simulink library "halout"  (R2021b)
settings: Solver=VariableStepAuto  StartTime=0.0  StopTime=10.0  RelTol=1e-3
undefined symbols (not defined in the file): C_TASK_5MS_S, FALSE, KHAL_CAN1TxReq_flg, KHAL_CAN2TxReq_flg, KHAL_CAN3FD3VCU1toNIDECTxReq_flg, KHAL_CAN3FD3VCU1TxReq_flg, KHAL_CAN3FD3VCU2E2E_flg, KHAL_CAN3FD3VCU2toNIDECE2E_flg, KHAL_CAN3FD3VCU2toNIDECTxReq_flg, KHAL_CAN3FD3VCU2TxReq_flg, KHAL_CAN3TxReq_flg, KHAL_CAN4FD4CE1000E2E_flg, KHAL_CAN4FD4CE1000TxReq_flg, KHAL_CAN4TxReq_flg, KHAL_CAN5TxReq_flg, KHAL_CAN7TxReq_flg, ONE_INT, TRUE, ZERO_INT
libraries: FVT_lib x258, simulink x115
(part 6 of 17)

== system halout/HAL_OUT/CAN3/FD3_VCU1_toNIDEC_0x116 ==
  BSCP_outputs : Inport  OutDataTypeStr=Bus: BSCP_outputs
  BOUTP_outputs : Inport  Port=2  OutDataTypeStr=Bus: BOUTP_outputs
  ActiveDischReqtoNidec : Subsystem
  CSVCU1toNidec : Subsystem
  CoastDwModeStaChktoNidec : Subsystem
  DCDCEnaReqtoNidec : Subsystem
  DCDCVoltSetpointtoNidec : Subsystem
  DemoModeStaChktoNidec : Subsystem
  DrSeatStatoNidec : Subsystem
  DynoModeStaChktoNidec : Subsystem
  FrActvDmpDisabReqtoNidec : Subsystem
  FrMCUEnaReqtoNidec : Subsystem
  Ground{,1..6} (7 alike) : Ground
  HVBatCnctReqtoNidec : Subsystem
  HVSysReadyToChargetoNidec : Subsystem
  LVChrgFuncStaChktoNidec : Subsystem
  MSACrlStatoNidec : Subsystem
  PrkReqtoNidec : Subsystem
  PwrStatoNidec : Subsystem
  RCVCU1toNidec : Subsystem
  RrActvDmpDisabReqtoNidec : Subsystem
  RrMCUEnaReqtoNidec : Subsystem
  ShiftGearPosntoNidec : Subsystem
  bus_creator : BusCreator  Inputs=20  OutDataTypeStr=Bus: DT_CAN3_SG_FD3_VCU1_toNIDEC  NonVirtualBus=on
  bus_selector : BusSelector  OutputSignals=VOUTP_ActiveDischargeReq_flg
  bus_selector1 : BusSelector  OutputSignals=VOUTP_DCDCEnaReq_flg
  bus_selector10 : BusSelector  OutputSignals=VOUTP_RrActvDmpDisabReq_flg
  bus_selector11 : BusSelector  OutputSignals=VOUTP_RrMCUEnaReq_flg
  bus_selector12 : BusSelector  OutputSignals=VOUTP_ShiftGearPosn_enum
  bus_selector2 : BusSelector  OutputSignals=VOUTP_DCDCVoltSetpoint_V
  bus_selector3 : BusSelector  OutputSignals=VOUTP_DrSeatSta_enum
  bus_selector4 : BusSelector  OutputSignals=VOUTP_FrActvDmpDisabReq_flg
  bus_selector5 : BusSelector  OutputSignals=VOUTP_FrMCUEnaReq_flg
  bus_selector6 : BusSelector  OutputSignals=VOUTP_HVBatCnctReq_flg
  bus_selector7 : BusSelector  OutputSignals=VOUTP_HVSysReadyToCharge_enum
  bus_selector8 : BusSelector  OutputSignals=VOUTP_MSACtrlSta_enum
  bus_selector9 : BusSelector  OutputSignals=VOUTP_PowerSta_enum
  FD3_VCU1_toNIDEC : Outport
  wires:
  BSCP_outputs/1 -> [BSCP_outputs]
  BOUTP_outputs/1 -> [BOUTP_outputs]
  [CAN3_ActiveDischReq_toNidec] -> bus_creator/1  "CAN3_ActiveDischReq_toNidec"
  [CAN3_CS_VCU1_toNidec] -> bus_creator/2  "CAN3_CS_VCU1_toNidec"
  [CAN3_CoastDwModeStaChk_toNidec] -> bus_creator/3  "CAN3_CoastDwModeStaChk_toNidec"
  [CAN3_DCDCEnaReq_toNidec] -> bus_creator/4  "CAN3_DCDCEnaReq_toNidec"
  [CAN3_DCDCVoltSetpoint_toNidec] -> bus_creator/5  "CAN3_DCDCVoltSetpoint_toNidec"
  [CAN3_DemoModeStaChk_toNidec] -> bus_creator/6  "CAN3_DemoModeStaChk_toNidec"
  [CAN3_Dr_SeatSta_toNidec] -> bus_creator/7  "CAN3_Dr_SeatSta_toNidec"
  [CAN3_DynoModeStaChk_toNidec] -> bus_creator/8  "CAN3_DynoModeStaChk_toNidec"
  [CAN3_Fr_ActvDmpDisabReq_toNidec] -> bus_creator/9  "CAN3_Fr_ActvDmpDisabReq_toNidec"
  [CAN3_Fr_MCUEnaReq_toNidec] -> bus_creator/10  "CAN3_Fr_MCUEnaReq_toNidec"
  [CAN3_HVBatCnctReq_toNidec] -> bus_creator/11  "CAN3_HVBatCnctReq_toNidec"
  [CAN3_HVSysReadyToCharge_toNidec] -> bus_creator/12  "CAN3_HVSysReadyToCharge_toNidec"
  [CAN3_LVChrgFuncStaChk_toNidec] -> bus_creator/13  "CAN3_LVChrgFuncStaChk_toNidec"
  [CAN3_MSA_Crl_Sta_toNidec] -> bus_creator/14  "CAN3_MSA_Crl_Sta_toNidec"
  [CAN3_PrkReq_toNidec] -> bus_creator/15  "CAN3_PrkReq_toNidec"
  [CAN3_PwrSta_toNidec] -> bus_creator/16  "CAN3_PwrSta_toNidec"
  [CAN3_RC_VCU1_toNidec] -> bus_creator/17  "CAN3_RC_VCU1_toNidec"
  [CAN3_Rr_ActvDmpDisabReq_toNidec] -> bus_creator/18  "CAN3_Rr_ActvDmpDisabReq_toNidec"
  [CAN3_Rr_MCUEnaReq_toNidec] -> bus_creator/19  "CAN3_Rr_MCUEnaReq_toNidec"
  [CAN3_ShiftGearPosn_toNidec] -> bus_creator/20  "CAN3_ShiftGearPosn_toNidec"
  bus_creator/1 -> FD3_VCU1_toNIDEC/1
  ActiveDischReqtoNidec/1(CAN3_ActiveDischReq_toNidec) -> [CAN3_ActiveDischReq_toNidec]
  CSVCU1toNidec/1(CAN3_CS_VCU1_toNidec) -> [CAN3_CS_VCU1_toNidec]
  CoastDwModeStaChktoNidec/1(CAN3_CoastDwModeStaChk_toNidec) -> [CAN3_CoastDwModeStaChk_toNidec]
  DCDCEnaReqtoNidec/1(CAN3_DCDCEnaReq_toNidec) -> [CAN3_DCDCEnaReq_toNidec]
  DCDCVoltSetpointtoNidec/1(CAN3_DCDCVoltSetpoint_toNidec) -> [CAN3_DCDCVoltSetpoint_toNidec]
  DemoModeStaChktoNidec/1(CAN3_DemoModeStaChk_toNidec) -> [CAN3_DemoModeStaChk_toNidec]
  DrSeatStatoNidec/1(CAN3_Dr_SeatSta_toNidec) -> [CAN3_Dr_SeatSta_toNidec]
  DynoModeStaChktoNidec/1(CAN3_DynoModeStaChk_toNidec) -> [CAN3_DynoModeStaChk_toNidec]
  FrActvDmpDisabReqtoNidec/1(CAN3_Fr_ActvDmpDisabReq_toNidec) -> [CAN3_Fr_ActvDmpDisabReq_toNidec]
  FrMCUEnaReqtoNidec/1(CAN3_Fr_MCUEnaReq_toNidec) -> [CAN3_Fr_MCUEnaReq_toNidec]
  HVBatCnctReqtoNidec/1(CAN3_HVBatCnctReq_toNidec) -> [CAN3_HVBatCnctReq_toNidec]
  HVSysReadyToChargetoNidec/1(CAN3_HVSysReadyToCharge_toNidec) -> [CAN3_HVSysReadyToCharge_toNidec]
  LVChrgFuncStaChktoNidec/1(CAN3_LVChrgFuncStaChk_toNidec) -> [CAN3_LVChrgFuncStaChk_toNidec]
  MSACrlStatoNidec/1(CAN3_MSA_Crl_Sta_toNidec) -> [CAN3_MSA_Crl_Sta_toNidec]
  PrkReqtoNidec/1(CAN3_PrkReq_toNidec) -> [CAN3_PrkReq_toNidec]
  PwrStatoNidec/1(CAN3_PwrSta_toNidec) -> [CAN3_PwrSta_toNidec]
  RCVCU1toNidec/1(CAN3_RC_VCU1_toNidec) -> [CAN3_RC_VCU1_toNidec]
  RrActvDmpDisabReqtoNidec/1(CAN3_Rr_ActvDmpDisabReq_toNidec) -> [CAN3_Rr_ActvDmpDisabReq_toNidec]
  RrMCUEnaReqtoNidec/1(CAN3_Rr_MCUEnaReq_toNidec) -> [CAN3_Rr_MCUEnaReq_toNidec]
  ShiftGearPosntoNidec/1(CAN3_ShiftGearPosn_toNidec) -> [CAN3_ShiftGearPosn_toNidec]
  bus_selector/1 -> ActiveDischReqtoNidec/1(ActiveDischReqtoNidec)  "<VOUTP_ActiveDischargeReq_flg>"
  [BOUTP_outputs] -> bus_selector/1
  Ground/1 -> CSVCU1toNidec/1(CSVCU1toNidec)
  Ground1/1 -> CoastDwModeStaChktoNidec/1(CoastDwModeStaChktoNidec)
  bus_selector1/1 -> DCDCEnaReqtoNidec/1(DCDCEnaReqtoNidec)  "<VOUTP_DCDCEnaReq_flg>"
  [BOUTP_outputs] -> bus_selector1/1
  bus_selector2/1 -> DCDCVoltSetpointtoNidec/1(DCDCVoltSetpointtoNidec)  "<VOUTP_DCDCVoltSetpoint_V>"
  [BOUTP_outputs] -> bus_selector2/1
  Ground2/1 -> DemoModeStaChktoNidec/1(DemoModeStaChktoNidec)
  bus_selector3/1 -> DrSeatStatoNidec/1(DrSeatStatoNidec)  "<VOUTP_DrSeatSta_enum>"
  [BOUTP_outputs] -> bus_selector3/1
  Ground3/1 -> DynoModeStaChktoNidec/1(DynoModeStaChktoNidec)
  bus_selector4/1 -> FrActvDmpDisabReqtoNidec/1(FrActvDmpDisabReqtoNidec)  "<VOUTP_FrActvDmpDisabReq_flg>"
  [BOUTP_outputs] -> bus_selector4/1
  bus_selector5/1 -> FrMCUEnaReqtoNidec/1(FrMCUEnaReqtoNidec)  "<VOUTP_FrMCUEnaReq_flg>"
  [BOUTP_outputs] -> bus_selector5/1
  bus_selector6/1 -> HVBatCnctReqtoNidec/1(HVBatCnctReqtoNidec)  "<VOUTP_HVBatCnctReq_flg>"
  [BOUTP_outputs] -> bus_selector6/1
  bus_selector7/1 -> HVSysReadyToChargetoNidec/1(HVSysReadyToChargetoNidec)  "<VOUTP_HVSysReadyToCharge_enum>"
  [BOUTP_outputs] -> bus_selector7/1
  Ground4/1 -> LVChrgFuncStaChktoNidec/1(LVChrgFuncStaChktoNidec)
  bus_selector8/1 -> MSACrlStatoNidec/1(MSACrlStatoNidec)  "<VOUTP_MSACtrlSta_enum>"
  [BOUTP_outputs] -> bus_selector8/1
  Ground5/1 -> PrkReqtoNidec/1(PrkReqtoNidec)
  bus_selector9/1 -> PwrStatoNidec/1(PwrStatoNidec)  "<VOUTP_PowerSta_enum>"
  [BOUTP_outputs] -> bus_selector9/1
  Ground6/1 -> RCVCU1toNidec/1(RCVCU1toNidec)
  bus_selector10/1 -> RrActvDmpDisabReqtoNidec/1(RrActvDmpDisabReqtoNidec)  "<VOUTP_RrActvDmpDisabReq_flg>"
  [BOUTP_outputs] -> bus_selector10/1
  bus_selector11/1 -> RrMCUEnaReqtoNidec/1(RrMCUEnaReqtoNidec)  "<VOUTP_RrMCUEnaReq_flg>"
  [BOUTP_outputs] -> bus_selector11/1
  bus_selector12/1 -> ShiftGearPosntoNidec/1(ShiftGearPosntoNidec)  "<VOUTP_ShiftGearPosn_enum>"
  [BOUTP_outputs] -> bus_selector12/1

== system halout/HAL_OUT/CAN3/FD3_VCU1_toNIDEC_Tx ==
  TxReq : Inport
  BSCP_outputs : Inport  Port=2  OutDataTypeStr=Bus: BSCP_outputs
  BOUTP_outputs : Inport  Port=3  OutDataTypeStr=Bus: BOUTP_outputs
  Chart : Stateflow chart  AncestorBlock=haloutREF/HAL_OUT/CAN3/FD3_VCU1_toNIDEC_Tx/Chart  TreatAsAtomicUnit=on
  Constant : Constant  Value=C_TASK_5MS_S
  Constant3 : Constant  Value=CycleTime
  Data Type Conversion : DataTypeConversion  OutDataTypeStr=uint16
  Data Type Conversion1 : DataTypeConversion  OutDataTypeStr=uint8
  Divide : Product  Inputs=*/
  Gain : Gain  Gain=0.001
  Ground{,1..6} (7 alike) : Ground
  OR : Logic  Operator=OR  Inputs=20  AllPortsSameDT=off  OutDataTypeStr=boolean
  bus_selector : BusSelector  OutputSignals=VOUTP_ActiveDischargeReq_flg
  bus_selector1 : BusSelector  OutputSignals=VOUTP_DCDCEnaReq_flg
  bus_selector10 : BusSelector  OutputSignals=VOUTP_RrActvDmpDisabReq_flg
  bus_selector11 : BusSelector  OutputSignals=VOUTP_RrMCUEnaReq_flg
  bus_selector12 : BusSelector  OutputSignals=VOUTP_ShiftGearPosn_enum
  bus_selector2 : BusSelector  OutputSignals=VOUTP_DCDCVoltSetpoint_V
  bus_selector3 : BusSelector  OutputSignals=VOUTP_DrSeatSta_enum
  bus_selector4 : BusSelector  OutputSignals=VOUTP_FrActvDmpDisabReq_flg
  bus_selector5 : BusSelector  OutputSignals=VOUTP_FrMCUEnaReq_flg
  bus_selector6 : BusSelector  OutputSignals=VOUTP_HVBatCnctReq_flg
  bus_selector7 : BusSelector  OutputSignals=VOUTP_HVSysReadyToCharge_enum
  bus_selector8 : BusSelector  OutputSignals=VOUTP_MSACtrlSta_enum
  bus_selector9 : BusSelector  OutputSignals=VOUTP_PowerSta_enum
  convert_out : FVT_lib/hal/convert_out  gain=0.0235  offset=12
  detect_change{,1..12} (13 alike) : simulink/Logic and Bit Operations/Detect Change  vinit=0  OutDataTypeStr=boolean
  TxTrigger : Outport
  wires:
  Data Type Conversion/1 -> Chart/3(CycleCnt)
  TxReq/1 -> Chart/1(TxReq)
  [EventReq_flg] -> Chart/2(EventReq)
  Constant/1 -> Divide/2
  Divide/1 -> Data Type Conversion/1
  Chart/1(TxTrigger) -> TxTrigger/1
  Gain/1 -> Divide/1
  Constant3/1 -> Gain/1
  BSCP_outputs/1 -> [BSCP_outputs]
  BOUTP_outputs/1 -> [BOUTP_outputs]
  OR/1 -> [EventReq_flg]
  detect_change/1 -> OR/1
  bus_selector/1 -> detect_change/1  "<VOUTP_ActiveDischargeReq_flg>"
  [BOUTP_outputs] -> bus_selector/1
  Ground/1 -> OR/2
  Ground1/1 -> OR/3
  detect_change1/1 -> OR/4
  bus_selector1/1 -> detect_change1/1  "<VOUTP_DCDCEnaReq_flg>"
  [BOUTP_outputs] -> bus_selector1/1
  detect_change2/1 -> OR/5
  Data Type Conversion1/1 -> detect_change2/1
  convert_out/1 -> Data Type Conversion1/1
  bus_selector2/1 -> convert_out/1  "<VOUTP_DCDCVoltSetpoint_V>"
  [BOUTP_outputs] -> bus_selector2/1
  Ground2/1 -> OR/6
  detect_change3/1 -> OR/7
  bus_selector3/1 -> detect_change3/1  "<VOUTP_DrSeatSta_enum>"
  [BOUTP_outputs] -> bus_selector3/1
  Ground3/1 -> OR/8
  detect_change4/1 -> OR/9
  bus_selector4/1 -> detect_change4/1  "<VOUTP_FrActvDmpDisabReq_flg>"
  [BOUTP_outputs] -> bus_selector4/1
  detect_change5/1 -> OR/10
  bus_selector5/1 -> detect_change5/1  "<VOUTP_FrMCUEnaReq_flg>"
  [BOUTP_outputs] -> bus_selector5/1
  detect_change6/1 -> OR/11
  bus_selector6/1 -> detect_change6/1  "<VOUTP_HVBatCnctReq_flg>"
  [BOUTP_outputs] -> bus_selector6/1
  detect_change7/1 -> OR/12
  bus_selector7/1 -> detect_change7/1  "<VOUTP_HVSysReadyToCharge_enum>"
  [BOUTP_outputs] -> bus_selector7/1
  Ground4/1 -> OR/13
  detect_change8/1 -> OR/14
  bus_selector8/1 -> detect_change8/1  "<VOUTP_MSACtrlSta_enum>"
  [BOUTP_outputs] -> bus_selector8/1
  Ground5/1 -> OR/15
  detect_change9/1 -> OR/16
  bus_selector9/1 -> detect_change9/1  "<VOUTP_PowerSta_enum>"
  [BOUTP_outputs] -> bus_selector9/1
  Ground6/1 -> OR/17
  detect_change10/1 -> OR/18
  bus_selector10/1 -> detect_change10/1  "<VOUTP_RrActvDmpDisabReq_flg>"
  [BOUTP_outputs] -> bus_selector10/1
  detect_change11/1 -> OR/19
  bus_selector11/1 -> detect_change11/1  "<VOUTP_RrMCUEnaReq_flg>"
  [BOUTP_outputs] -> bus_selector11/1
  detect_change12/1 -> OR/20
  bus_selector12/1 -> detect_change12/1  "<VOUTP_ShiftGearPosn_enum>"
  [BOUTP_outputs] -> bus_selector12/1

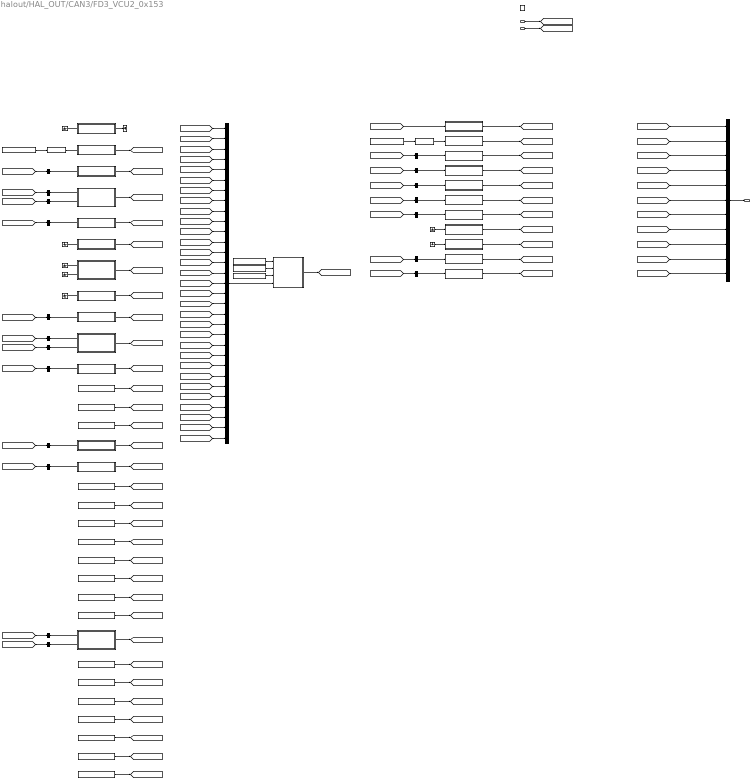
== system halout/HAL_OUT/CAN3/FD3_VCU2_0x153 ==
  BSCP_outputs : Inport  OutDataTypeStr=Bus: BSCP_outputs
  BOUTP_outputs : Inport  Port=2  OutDataTypeStr=Bus: BOUTP_outputs
  Trigger : TriggerPort  TriggerType=function-call  VariantControl=(inherit)
  Byte_0 : Subsystem
  Byte_1 : Subsystem
  Byte_10 : Subsystem
  Byte_{11..13,16..23,25..31} (18 alike) : Constant  Value=ZERO_INT
  Byte_14 : Subsystem
  Byte_15 : Subsystem
  Byte_2 : Subsystem
  Byte_24 : Subsystem
  Byte_3 : Subsystem
  Byte_4 : Subsystem
  Byte_5 : Subsystem
  Byte_6 : Subsystem
  Byte_7 : Subsystem
  Byte_8 : Subsystem
  Byte_9 : Subsystem
  CRC8_IfAction_Tx : Subsystem  AncestorBlock=FVT_lib/hal/CRC8_IfAction_Tx
      mask help: MeasumentTrigerEvent
      mask Display: fprintf('CRC8_IfAction');
  CSVCU2CAN1 : Subsystem
  Constant : Constant  Value=KHAL_CAN3FD3VCU2E2E_flg
  Constant1 : Constant  Value=0x40
  Constant2 : Constant  Value=0x24
  Constant3 : Constant  Value=KHAL_CAN3FD3VCU2E2E_flg
  Constant4 : Constant  Value=KHAL_CAN3FD3VCU2E2E_flg
  Ground{,1..6} (7 alike) : Ground
  Mux2 : Mux  Inputs=31
  RCVCU2CAN1 : Subsystem
  RollingCounter_IfAction : FVT_lib/hal/RollingCounter_IfAction
  RollingCounter_IfAction1 : FVT_lib/hal/RollingCounter_IfAction
  RrActvDmpDisabReq : Subsystem
  RrIdcMax : Subsystem
  RrIdcMin : Subsystem
  RrMCUEnaReq : Subsystem
  RrTMTqReq : Subsystem
  RrTorqMax : Subsystem
  RrTorqMin : Subsystem
  RrUdcMax : Subsystem
  RrUdcMin : Subsystem
  Terminator : Terminator
  bus_creator : BusCreator  Inputs=11  OutDataTypeStr=Bus: DT_CAN3_SG_FD3_VCU2  NonVirtualBus=on
  bus_selector : BusSelector  OutputSignals=VOUTP_RrIdcMax_A
  bus_selector1 : BusSelector  OutputSignals=VOUTP_RrIdcMax_A
  bus_selector10 : BusSelector  OutputSignals=VOUTP_RrActvDmpDisabReq_flg
  bus_selector11 : BusSelector  OutputSignals=VOUTP_RrMCUEnaReq_flg
  bus_selector12 : BusSelector  OutputSignals=VOUTP_RrActvDmpDisabReq_flg
  bus_selector13 : BusSelector  OutputSignals=VOUTP_RrIdcMax_A
  bus_selector14 : BusSelector  OutputSignals=VOUTP_RrIdcMin_A
  bus_selector15 : BusSelector  OutputSignals=VOUTP_RrMCUEnaReq_flg
  bus_selector16 : BusSelector  OutputSignals=VOUTP_RrTMTqReq_Nm
  bus_selector17 : BusSelector  OutputSignals=VOUTP_RrUdcMax_V
  bus_selector18 : BusSelector  OutputSignals=VOUTP_RrUdcMin_V
  bus_selector2 : BusSelector  OutputSignals=VOUTP_RrIdcMin_A
  bus_selector3 : BusSelector  OutputSignals=VOUTP_RrIdcMin_A
  bus_selector4 : BusSelector  OutputSignals=VOUTP_RrUdcMax_V
  bus_selector5 : BusSelector  OutputSignals=VOUTP_RrUdcMax_V
  bus_selector6 : BusSelector  OutputSignals=VOUTP_RrUdcMin_V
  bus_selector7 : BusSelector  OutputSignals=VOUTP_RrUdcMin_V
  bus_selector8 : BusSelector  OutputSignals=VOUTP_RrTMTqReq_Nm
  bus_selector9 : BusSelector  OutputSignals=VOUTP_RrTMTqReq_Nm
  FD3_VCU2 : Outport
  wires:
  BSCP_outputs/1 -> [BSCP_outputs]
  BOUTP_outputs/1 -> [BOUTP_outputs]
  [CAN3_CS_VCU2_CAN1] -> bus_creator/1  "CAN3_CS_VCU2_CAN1"
  [CAN3_RC_VCU2_CAN1] -> bus_creator/2  "CAN3_RC_VCU2_CAN1"
  [CAN3_Rr_ActvDmpDisabReq] -> bus_creator/3  "CAN3_Rr_ActvDmpDisabReq"
  [CAN3_Rr_IdcMax] -> bus_creator/4  "CAN3_Rr_IdcMax"
  [CAN3_Rr_IdcMin] -> bus_creator/5  "CAN3_Rr_IdcMin"
  [CAN3_Rr_MCUEnaReq] -> bus_creator/6  "CAN3_Rr_MCUEnaReq"
  [CAN3_Rr_TMTqReq] -> bus_creator/7  "CAN3_Rr_TMTqReq"
  [CAN3_Rr_TorqMax] -> bus_creator/8  "CAN3_Rr_TorqMax"
  [CAN3_Rr_TorqMin] -> bus_creator/9  "CAN3_Rr_TorqMin"
  [CAN3_Rr_UdcMax] -> bus_creator/10  "CAN3_Rr_UdcMax"
  [CAN3_Rr_UdcMin] -> bus_creator/11  "CAN3_Rr_UdcMin"
  bus_creator/1 -> FD3_VCU2/1
  CSVCU2CAN1/1(CAN3_CS_VCU2_CAN1) -> [CAN3_CS_VCU2_CAN1]
  RCVCU2CAN1/1(CAN3_RC_VCU2_CAN1) -> [CAN3_RC_VCU2_CAN1]
  RrActvDmpDisabReq/1(CAN3_Rr_ActvDmpDisabReq) -> [CAN3_Rr_ActvDmpDisabReq]
  RrIdcMax/1(CAN3_Rr_IdcMax) -> [CAN3_Rr_IdcMax]
  RrIdcMin/1(CAN3_Rr_IdcMin) -> [CAN3_Rr_IdcMin]
  RrMCUEnaReq/1(CAN3_Rr_MCUEnaReq) -> [CAN3_Rr_MCUEnaReq]
  RrTMTqReq/1(CAN3_Rr_TMTqReq) -> [CAN3_Rr_TMTqReq]
  RrTorqMax/1(CAN3_Rr_TorqMax) -> [CAN3_Rr_TorqMax]
  RrTorqMin/1(CAN3_Rr_TorqMin) -> [CAN3_Rr_TorqMin]
  RrUdcMax/1(CAN3_Rr_UdcMax) -> [CAN3_Rr_UdcMax]
  RrUdcMin/1(CAN3_Rr_UdcMin) -> [CAN3_Rr_UdcMin]
  Byte_0/1(Byte_0) -> Terminator/1
  Byte_1/1(Byte_1) -> [Byte_1]
  Byte_2/1(Byte_2) -> [Byte_2]
  Byte_3/1(Byte_3) -> [Byte_3]
  Byte_4/1(Byte_4) -> [Byte_4]
  Byte_5/1(Byte_5) -> [Byte_5]
  Byte_6/1(Byte_6) -> [Byte_6]
  Byte_7/1(Byte_7) -> [Byte_7]
  Byte_8/1(Byte_8) -> [Byte_8]
  Byte_9/1(Byte_9) -> [Byte_9]
  Byte_10/1(Byte_10) -> [Byte_10]
  Byte_11/1 -> [Byte_11]
  Byte_12/1 -> [Byte_12]
  Byte_13/1 -> [Byte_13]
  Byte_14/1(Byte_14) -> [Byte_14]
  Byte_15/1(Byte_15) -> [Byte_15]
  Byte_16/1 -> [Byte_16]
  Byte_17/1 -> [Byte_17]
  Byte_18/1 -> [Byte_18]
  Byte_19/1 -> [Byte_19]
  Byte_20/1 -> [Byte_20]
  Byte_21/1 -> [Byte_21]
  Byte_22/1 -> [Byte_22]
  Byte_23/1 -> [Byte_23]
  Byte_24/1(Byte_24) -> [Byte_24]
  Byte_25/1 -> [Byte_25]
  Byte_26/1 -> [Byte_26]
  Byte_27/1 -> [Byte_27]
  Byte_28/1 -> [Byte_28]
  Byte_29/1 -> [Byte_29]
  Byte_30/1 -> [Byte_30]
  Byte_31/1 -> [Byte_31]
  Mux2/1 -> CRC8_IfAction_Tx/4(RawData)
  Constant/1 -> CRC8_IfAction_Tx/1(CAN_E2E_flg)
  Constant1/1 -> CRC8_IfAction_Tx/2(DataID1)
  Constant2/1 -> CRC8_IfAction_Tx/3(DataID2)
  CRC8_IfAction_Tx/1(CRC8) -> [CS_VCU2_CAN1]
  Ground/1 -> Byte_0/1(CS_VCU2_CAN1)
  [Byte_1] -> Mux2/1
  RollingCounter_IfAction/1 -> Byte_1/1(RC_VCU2_CAN1)
  Constant3/1 -> RollingCounter_IfAction/1
  [Byte_2] -> Mux2/2
  bus_selector/1 -> Byte_2/1(Rr_IdcMax)  "<VOUTP_RrIdcMax_A>"
  [BOUTP_outputs] -> bus_selector/1
  [Byte_3] -> Mux2/3
  bus_selector1/1 -> Byte_3/1(Rr_IdcMax)  "<VOUTP_RrIdcMax_A>"
  [BOUTP_outputs] -> bus_selector1/1
  bus_selector2/1 -> Byte_3/2(Rr_IdcMin)  "<VOUTP_RrIdcMin_A>"
  [BOUTP_outputs] -> bus_selector2/1
  [Byte_4] -> Mux2/4
  bus_selector3/1 -> Byte_4/1(Rr_IdcMin)  "<VOUTP_RrIdcMin_A>"
  [BOUTP_outputs] -> bus_selector3/1
  [Byte_5] -> Mux2/5
  Ground1/1 -> Byte_5/1(Rr_TorqMax)
  [Byte_6] -> Mux2/6
  Ground2/1 -> Byte_6/1(Rr_TorqMax)
  Ground3/1 -> Byte_6/2(Rr_TorqMin)
  [Byte_7] -> Mux2/7
  Ground4/1 -> Byte_7/1(Rr_TorqMin)
  [Byte_8] -> Mux2/8
  bus_selector4/1 -> Byte_8/1(Rr_UdcMax)  "<VOUTP_RrUdcMax_V>"
  [BOUTP_outputs] -> bus_selector4/1
  [Byte_9] -> Mux2/9
  bus_selector5/1 -> Byte_9/1(Rr_UdcMax)  "<VOUTP_RrUdcMax_V>"
  [BOUTP_outputs] -> bus_selector5/1
  bus_selector6/1 -> Byte_9/2(Rr_UdcMin)  "<VOUTP_RrUdcMin_V>"
  [BOUTP_outputs] -> bus_selector6/1
  [Byte_10] -> Mux2/10
  bus_selector7/1 -> Byte_10/1(Rr_UdcMin)  "<VOUTP_RrUdcMin_V>"
  [BOUTP_outputs] -> bus_selector7/1
  [Byte_11] -> Mux2/11
  [Byte_12] -> Mux2/12
  [Byte_13] -> Mux2/13
  [Byte_14] -> Mux2/14
  bus_selector8/1 -> Byte_14/1(Rr_TMTqReq)  "<VOUTP_RrTMTqReq_Nm>"
  [BOUTP_outputs] -> bus_selector8/1
  [Byte_15] -> Mux2/15
  bus_selector9/1 -> Byte_15/1(Rr_TMTqReq)  "<VOUTP_RrTMTqReq_Nm>"
  [BOUTP_outputs] -> bus_selector9/1
  [Byte_16] -> Mux2/16
  [Byte_17] -> Mux2/17
  [Byte_18] -> Mux2/18
  [Byte_19] -> Mux2/19
  [Byte_20] -> Mux2/20
  [Byte_21] -> Mux2/21
  [Byte_22] -> Mux2/22
  [Byte_23] -> Mux2/23
  [Byte_24] -> Mux2/24
  bus_selector10/1 -> Byte_24/1(Rr_ActvDmpDisabReq)  "<VOUTP_RrActvDmpDisabReq_flg>"
  [BOUTP_outputs] -> bus_selector10/1
  bus_selector11/1 -> Byte_24/2(Rr_MCUEnaReq)  "<VOUTP_RrMCUEnaReq_flg>"
  [BOUTP_outputs] -> bus_selector11/1
  [Byte_25] -> Mux2/25
  [Byte_26] -> Mux2/26
  [Byte_27] -> Mux2/27
  [Byte_28] -> Mux2/28
  [Byte_29] -> Mux2/29
  [Byte_30] -> Mux2/30
  [Byte_31] -> Mux2/31
  [CS_VCU2_CAN1] -> CSVCU2CAN1/1(CSVCU2CAN1)
  RollingCounter_IfAction1/1 -> RCVCU2CAN1/1(RCVCU2CAN1)
  Constant4/1 -> RollingCounter_IfAction1/1
  bus_selector12/1 -> RrActvDmpDisabReq/1(RrActvDmpDisabReq)  "<VOUTP_RrActvDmpDisabReq_flg>"
  [BOUTP_outputs] -> bus_selector12/1
  bus_selector13/1 -> RrIdcMax/1(RrIdcMax)  "<VOUTP_RrIdcMax_A>"
  [BOUTP_outputs] -> bus_selector13/1
  bus_selector14/1 -> RrIdcMin/1(RrIdcMin)  "<VOUTP_RrIdcMin_A>"
  [BOUTP_outputs] -> bus_selector14/1
  bus_selector15/1 -> RrMCUEnaReq/1(RrMCUEnaReq)  "<VOUTP_RrMCUEnaReq_flg>"
  [BOUTP_outputs] -> bus_selector15/1
  bus_selector16/1 -> RrTMTqReq/1(RrTMTqReq)  "<VOUTP_RrTMTqReq_Nm>"
  [BOUTP_outputs] -> bus_selector16/1
  Ground5/1 -> RrTorqMax/1(RrTorqMax)
  Ground6/1 -> RrTorqMin/1(RrTorqMin)
  bus_selector17/1 -> RrUdcMax/1(RrUdcMax)  "<VOUTP_RrUdcMax_V>"
  [BOUTP_outputs] -> bus_selector17/1
  bus_selector18/1 -> RrUdcMin/1(RrUdcMin)  "<VOUTP_RrUdcMin_V>"
  [BOUTP_outputs] -> bus_selector18/1

== system halout/HAL_OUT/CAN3/FD3_VCU2_Tx ==
  TxReq : Inport
  Chart : Stateflow chart  TreatAsAtomicUnit=on
  Constant : Constant  Value=C_TASK_5MS_S
  Constant3 : Constant  Value=CycleTime
  Data Type Conversion : DataTypeConversion  OutDataTypeStr=uint16
  Divide : Product  Inputs=*/
  Gain : Gain  Gain=0.001
  TxTrigger : Outport
  wires:
  Data Type Conversion/1 -> Chart/2(CycleCnt)
  Constant3/1 -> Gain/1
  Gain/1 -> Divide/1
  Chart/1(TxTrigger()) -> TxTrigger/1
  Divide/1 -> Data Type Conversion/1
  TxReq/1 -> Chart/1(TxReq)
  Constant/1 -> Divide/2

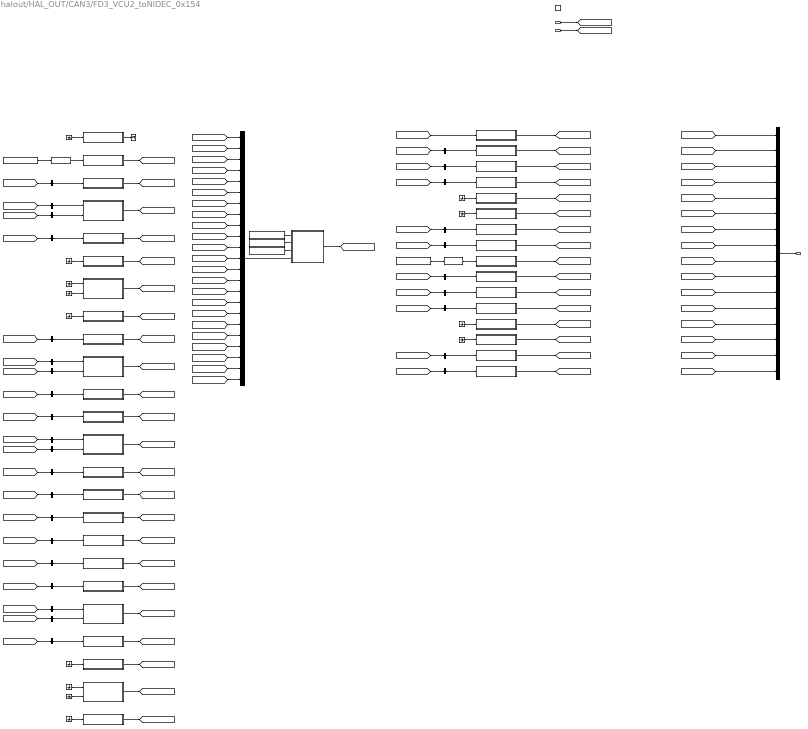
== system halout/HAL_OUT/CAN3/FD3_VCU2_toNIDEC_0x154 ==
  BSCP_outputs : Inport  OutDataTypeStr=Bus: BSCP_outputs
  BOUTP_outputs : Inport  Port=2  OutDataTypeStr=Bus: BOUTP_outputs
  Trigger : TriggerPort  TriggerType=function-call  VariantControl=(inherit)
  Byte_0 : Subsystem
  Byte_1 : Subsystem
  Byte_10 : Subsystem
  Byte_11 : Subsystem
  Byte_12 : Subsystem
  Byte_13 : Subsystem
  Byte_14 : Subsystem
  Byte_15 : Subsystem
  Byte_16 : Subsystem
  Byte_17 : Subsystem
  Byte_18 : Subsystem
  Byte_19 : Subsystem
  Byte_2 : Subsystem
  Byte_20 : Subsystem
  Byte_21 : Subsystem
  Byte_22 : Subsystem
  Byte_23 : Subsystem
  Byte_3 : Subsystem
  Byte_4 : Subsystem
  Byte_5 : Subsystem
  Byte_6 : Subsystem
  Byte_7 : Subsystem
  Byte_8 : Subsystem
  Byte_9 : Subsystem
  CRC8_IfAction_Tx : Subsystem  AncestorBlock=FVT_lib/hal/CRC8_IfAction_Tx
      mask help: MeasumentTrigerEvent
      mask Display: fprintf('CRC8_IfAction');
  CSVCU2CAN1toNidec : Subsystem
  Constant : Constant  Value=KHAL_CAN3FD3VCU2toNIDECE2E_flg
  Constant1 : Constant  Value=0x41
  Constant2 : Constant  Value=0x14
  Constant3 : Constant  Value=KHAL_CAN3FD3VCU2toNIDECE2E_flg
  Constant4 : Constant  Value=KHAL_CAN3FD3VCU2toNIDECE2E_flg
  FrIdcMaxtoNidec : Subsystem
  FrIdcMintoNidec : Subsystem
  FrTMTqReqtoNidec : Subsystem
  FrTorqMaxtoNidec : Subsystem
  FrTorqMintoNidec : Subsystem
  FrUdcMaxtoNidec : Subsystem
  FrUdcMintoNidec : Subsystem
  Ground{,1..12} (13 alike) : Ground
  Mux2 : Mux  Inputs=23
  RCVCU2CAN1toNidec : Subsystem
  RollingCounter_IfAction : FVT_lib/hal/RollingCounter_IfAction
  RollingCounter_IfAction1 : FVT_lib/hal/RollingCounter_IfAction
  RrIdcMaxtoNidec : Subsystem
  RrIdcMintoNidec : Subsystem
  RrTMTqReqtoNidec : Subsystem
  RrTorqMaxtoNidec : Subsystem
  RrTorqMintoNidec : Subsystem
  RrUdcMaxtoNidec : Subsystem
  RrUdcMintoNidec : Subsystem
  Terminator : Terminator
  bus_creator : BusCreator  Inputs=16  OutDataTypeStr=Bus: DT_CAN3_SG_FD3_VCU2_toNIDEC  NonVirtualBus=on
  bus_selector : BusSelector  OutputSignals=VOUTP_RrIdcMax_A
  bus_selector1 : BusSelector  OutputSignals=VOUTP_RrIdcMax_A
  bus_selector10 : BusSelector  OutputSignals=VOUTP_FrUdcMin_V
  bus_selector11 : BusSelector  OutputSignals=VOUTP_FrUdcMin_V
  bus_selector12 : BusSelector  OutputSignals=VOUTP_RrTMTqReq_Nm
  bus_selector13 : BusSelector  OutputSignals=VOUTP_RrTMTqReq_Nm
  bus_selector14 : BusSelector  OutputSignals=VOUTP_FrTMTqReq_Nm
  bus_selector15 : BusSelector  OutputSignals=VOUTP_FrTMTqReq_Nm
  bus_selector16 : BusSelector  OutputSignals=VOUTP_FrIdcMax_A
  bus_selector17 : BusSelector  OutputSignals=VOUTP_FrIdcMax_A
  bus_selector18 : BusSelector  OutputSignals=VOUTP_FrIdcMin_A
  bus_selector19 : BusSelector  OutputSignals=VOUTP_FrIdcMin_A
  bus_selector2 : BusSelector  OutputSignals=VOUTP_RrIdcMin_A
  bus_selector20 : BusSelector  OutputSignals=VOUTP_FrIdcMax_A
  bus_selector21 : BusSelector  OutputSignals=VOUTP_FrIdcMin_A
  bus_selector22 : BusSelector  OutputSignals=VOUTP_FrTMTqReq_Nm
  bus_selector23 : BusSelector  OutputSignals=VOUTP_FrUdcMax_V
  bus_selector24 : BusSelector  OutputSignals=VOUTP_FrUdcMin_V
  bus_selector25 : BusSelector  OutputSignals=VOUTP_RrIdcMax_A
  bus_selector26 : BusSelector  OutputSignals=VOUTP_RrIdcMin_A
  bus_selector27 : BusSelector  OutputSignals=VOUTP_RrTMTqReq_Nm
  bus_selector28 : BusSelector  OutputSignals=VOUTP_RrUdcMax_V
  bus_selector29 : BusSelector  OutputSignals=VOUTP_RrUdcMin_V
  bus_selector3 : BusSelector  OutputSignals=VOUTP_RrIdcMin_A
  bus_selector4 : BusSelector  OutputSignals=VOUTP_RrUdcMax_V
  bus_selector5 : BusSelector  OutputSignals=VOUTP_RrUdcMax_V
  bus_selector6 : BusSelector  OutputSignals=VOUTP_RrUdcMin_V
  bus_selector7 : BusSelector  OutputSignals=VOUTP_RrUdcMin_V
  bus_selector8 : BusSelector  OutputSignals=VOUTP_FrUdcMax_V
  bus_selector9 : BusSelector  OutputSignals=VOUTP_FrUdcMax_V
  FD3_VCU2_toNIDEC : Outport
  wires:
  BSCP_outputs/1 -> [BSCP_outputs]
  BOUTP_outputs/1 -> [BOUTP_outputs]
  [CAN3_CS_VCU2_CAN1_toNidec] -> bus_creator/1  "CAN3_CS_VCU2_CAN1_toNidec"
  [CAN3_Fr_IdcMax_toNidec] -> bus_creator/2  "CAN3_Fr_IdcMax_toNidec"
  [CAN3_Fr_IdcMin_toNidec] -> bus_creator/3  "CAN3_Fr_IdcMin_toNidec"
  [CAN3_Fr_TMTqReq_toNidec] -> bus_creator/4  "CAN3_Fr_TMTqReq_toNidec"
  [CAN3_Fr_TorqMax_toNidec] -> bus_creator/5  "CAN3_Fr_TorqMax_toNidec"
  [CAN3_Fr_TorqMin_toNidec] -> bus_creator/6  "CAN3_Fr_TorqMin_toNidec"
  [CAN3_Fr_UdcMax_toNidec] -> bus_creator/7  "CAN3_Fr_UdcMax_toNidec"
  [CAN3_Fr_UdcMin_toNidec] -> bus_creator/8  "CAN3_Fr_UdcMin_toNidec"
  [CAN3_RC_VCU2_CAN1_toNidec] -> bus_creator/9  "CAN3_RC_VCU2_CAN1_toNidec"
  [CAN3_Rr_IdcMax_toNidec] -> bus_creator/10  "CAN3_Rr_IdcMax_toNidec"
  [CAN3_Rr_IdcMin_toNidec] -> bus_creator/11  "CAN3_Rr_IdcMin_toNidec"
  [CAN3_Rr_TMTqReq_toNidec] -> bus_creator/12  "CAN3_Rr_TMTqReq_toNidec"
  [CAN3_Rr_TorqMax_toNidec] -> bus_creator/13  "CAN3_Rr_TorqMax_toNidec"
  [CAN3_Rr_TorqMin_toNidec] -> bus_creator/14  "CAN3_Rr_TorqMin_toNidec"
  [CAN3_Rr_UdcMax_toNidec] -> bus_creator/15  "CAN3_Rr_UdcMax_toNidec"
  [CAN3_Rr_UdcMin_toNidec] -> bus_creator/16  "CAN3_Rr_UdcMin_toNidec"
  bus_creator/1 -> FD3_VCU2_toNIDEC/1
  CSVCU2CAN1toNidec/1(CAN3_CS_VCU2_CAN1_toNidec) -> [CAN3_CS_VCU2_CAN1_toNidec]
  FrIdcMaxtoNidec/1(CAN3_Fr_IdcMax_toNidec) -> [CAN3_Fr_IdcMax_toNidec]
  FrIdcMintoNidec/1(CAN3_Fr_IdcMin_toNidec) -> [CAN3_Fr_IdcMin_toNidec]
  FrTMTqReqtoNidec/1(CAN3_Fr_TMTqReq_toNidec) -> [CAN3_Fr_TMTqReq_toNidec]
  FrTorqMaxtoNidec/1(CAN3_Fr_TorqMax_toNidec) -> [CAN3_Fr_TorqMax_toNidec]
  FrTorqMintoNidec/1(CAN3_Fr_TorqMin_toNidec) -> [CAN3_Fr_TorqMin_toNidec]
  FrUdcMaxtoNidec/1(CAN3_Fr_UdcMax_toNidec) -> [CAN3_Fr_UdcMax_toNidec]
  FrUdcMintoNidec/1(CAN3_Fr_UdcMin_toNidec) -> [CAN3_Fr_UdcMin_toNidec]
  RCVCU2CAN1toNidec/1(CAN3_RC_VCU2_CAN1_toNidec) -> [CAN3_RC_VCU2_CAN1_toNidec]
  RrIdcMaxtoNidec/1(CAN3_Rr_IdcMax_toNidec) -> [CAN3_Rr_IdcMax_toNidec]
  RrIdcMintoNidec/1(CAN3_Rr_IdcMin_toNidec) -> [CAN3_Rr_IdcMin_toNidec]
  RrTMTqReqtoNidec/1(CAN3_Rr_TMTqReq_toNidec) -> [CAN3_Rr_TMTqReq_toNidec]
  RrTorqMaxtoNidec/1(CAN3_Rr_TorqMax_toNidec) -> [CAN3_Rr_TorqMax_toNidec]
  RrTorqMintoNidec/1(CAN3_Rr_TorqMin_toNidec) -> [CAN3_Rr_TorqMin_toNidec]
  RrUdcMaxtoNidec/1(CAN3_Rr_UdcMax_toNidec) -> [CAN3_Rr_UdcMax_toNidec]
  RrUdcMintoNidec/1(CAN3_Rr_UdcMin_toNidec) -> [CAN3_Rr_UdcMin_toNidec]
  Byte_0/1(Byte_0) -> Terminator/1
  Byte_1/1(Byte_1) -> [Byte_1]
  Byte_2/1(Byte_2) -> [Byte_2]
  Byte_3/1(Byte_3) -> [Byte_3]
  Byte_4/1(Byte_4) -> [Byte_4]
  Byte_5/1(Byte_5) -> [Byte_5]
  Byte_6/1(Byte_6) -> [Byte_6]
  Byte_7/1(Byte_7) -> [Byte_7]
  Byte_8/1(Byte_8) -> [Byte_8]
  Byte_9/1(Byte_9) -> [Byte_9]
  Byte_10/1(Byte_10) -> [Byte_10]
  Byte_11/1(Byte_11) -> [Byte_11]
  Byte_12/1(Byte_12) -> [Byte_12]
  Byte_13/1(Byte_13) -> [Byte_13]
  Byte_14/1(Byte_14) -> [Byte_14]
  Byte_15/1(Byte_15) -> [Byte_15]
  Byte_16/1(Byte_16) -> [Byte_16]
  Byte_17/1(Byte_17) -> [Byte_17]
  Byte_18/1(Byte_18) -> [Byte_18]
  Byte_19/1(Byte_19) -> [Byte_19]
  Byte_20/1(Byte_20) -> [Byte_20]
  Byte_21/1(Byte_21) -> [Byte_21]
  Byte_22/1(Byte_22) -> [Byte_22]
  Byte_23/1(Byte_23) -> [Byte_23]
  Mux2/1 -> CRC8_IfAction_Tx/4(RawData)
  Constant/1 -> CRC8_IfAction_Tx/1(CAN_E2E_flg)
  Constant1/1 -> CRC8_IfAction_Tx/2(DataID1)
  Constant2/1 -> CRC8_IfAction_Tx/3(DataID2)
  CRC8_IfAction_Tx/1(CRC8) -> [CS_VCU2_CAN1_toNidec]
  Ground/1 -> Byte_0/1(CS_VCU2_CAN1_toNidec)
  [Byte_1] -> Mux2/1
  RollingCounter_IfAction/1 -> Byte_1/1(RC_VCU2_CAN1_toNidec)
  Constant3/1 -> RollingCounter_IfAction/1
  [Byte_2] -> Mux2/2
  bus_selector/1 -> Byte_2/1(Rr_IdcMax_toNidec)  "<VOUTP_RrIdcMax_A>"
  [BOUTP_outputs] -> bus_selector/1
  [Byte_3] -> Mux2/3
  bus_selector1/1 -> Byte_3/1(Rr_IdcMax_toNidec)  "<VOUTP_RrIdcMax_A>"
  [BOUTP_outputs] -> bus_selector1/1
  bus_selector2/1 -> Byte_3/2(Rr_IdcMin_toNidec)  "<VOUTP_RrIdcMin_A>"
  [BOUTP_outputs] -> bus_selector2/1
  [Byte_4] -> Mux2/4
  bus_selector3/1 -> Byte_4/1(Rr_IdcMin_toNidec)  "<VOUTP_RrIdcMin_A>"
  [BOUTP_outputs] -> bus_selector3/1
  [Byte_5] -> Mux2/5
  Ground1/1 -> Byte_5/1(Rr_TorqMax_toNidec)
  [Byte_6] -> Mux2/6
  Ground2/1 -> Byte_6/1(Rr_TorqMax_toNidec)
  Ground3/1 -> Byte_6/2(Rr_TorqMin_toNidec)
  [Byte_7] -> Mux2/7
  Ground4/1 -> Byte_7/1(Rr_TorqMin_toNidec)
  [Byte_8] -> Mux2/8
  bus_selector4/1 -> Byte_8/1(Rr_UdcMax_toNidec)  "<VOUTP_RrUdcMax_V>"
  [BOUTP_outputs] -> bus_selector4/1
  [Byte_9] -> Mux2/9
  bus_selector5/1 -> Byte_9/1(Rr_UdcMax_toNidec)  "<VOUTP_RrUdcMax_V>"
  [BOUTP_outputs] -> bus_selector5/1
  bus_selector6/1 -> Byte_9/2(Rr_UdcMin_toNidec)  "<VOUTP_RrUdcMin_V>"
  [BOUTP_outputs] -> bus_selector6/1
  [Byte_10] -> Mux2/10
  bus_selector7/1 -> Byte_10/1(Rr_UdcMin_toNidec)  "<VOUTP_RrUdcMin_V>"
  [BOUTP_outputs] -> bus_selector7/1
  [Byte_11] -> Mux2/11
  bus_selector8/1 -> Byte_11/1(Fr_UdcMax_toNidec)  "<VOUTP_FrUdcMax_V>"
  [BOUTP_outputs] -> bus_selector8/1
  [Byte_12] -> Mux2/12
  bus_selector9/1 -> Byte_12/1(Fr_UdcMax_toNidec)  "<VOUTP_FrUdcMax_V>"
  [BOUTP_outputs] -> bus_selector9/1
  bus_selector10/1 -> Byte_12/2(Fr_UdcMin_toNidec)  "<VOUTP_FrUdcMin_V>"
  [BOUTP_outputs] -> bus_selector10/1
  [Byte_13] -> Mux2/13
  bus_selector11/1 -> Byte_13/1(Fr_UdcMin_toNidec)  "<VOUTP_FrUdcMin_V>"
  [BOUTP_outputs] -> bus_selector11/1
  [Byte_14] -> Mux2/14
  bus_selector12/1 -> Byte_14/1(Rr_TMTqReq_toNidec)  "<VOUTP_RrTMTqReq_Nm>"
  [BOUTP_outputs] -> bus_selector12/1
  [Byte_15] -> Mux2/15
  bus_selector13/1 -> Byte_15/1(Rr_TMTqReq_toNidec)  "<VOUTP_RrTMTqReq_Nm>"
  [BOUTP_outputs] -> bus_selector13/1
  [Byte_16] -> Mux2/16
  bus_selector14/1 -> Byte_16/1(Fr_TMTqReq_toNidec)  "<VOUTP_FrTMTqReq_Nm>"
  [BOUTP_outputs] -> bus_selector14/1
  [Byte_17] -> Mux2/17
  bus_selector15/1 -> Byte_17/1(Fr_TMTqReq_toNidec)  "<VOUTP_FrTMTqReq_Nm>"
  [BOUTP_outputs] -> bus_selector15/1
  [Byte_18] -> Mux2/18
  bus_selector16/1 -> Byte_18/1(Fr_IdcMax_toNidec)  "<VOUTP_FrIdcMax_A>"
  [BOUTP_outputs] -> bus_selector16/1
  [Byte_19] -> Mux2/19
  bus_selector17/1 -> Byte_19/1(Fr_IdcMax_toNidec)  "<VOUTP_FrIdcMax_A>"
  [BOUTP_outputs] -> bus_selector17/1
  bus_selector18/1 -> Byte_19/2(Fr_IdcMin_toNidec)  "<VOUTP_FrIdcMin_A>"
  [BOUTP_outputs] -> bus_selector18/1
  [Byte_20] -> Mux2/20
  bus_selector19/1 -> Byte_20/1(Fr_IdcMin_toNidec)  "<VOUTP_FrIdcMin_A>"
  [BOUTP_outputs] -> bus_selector19/1
  [Byte_21] -> Mux2/21
  Ground5/1 -> Byte_21/1(Fr_TorqMax_toNidec)
  [Byte_22] -> Mux2/22
  Ground6/1 -> Byte_22/1(Fr_TorqMax_toNidec)
  Ground7/1 -> Byte_22/2(Fr_TorqMin_toNidec)
  [Byte_23] -> Mux2/23
  Ground8/1 -> Byte_23/1(Fr_TorqMin_toNidec)
  [CS_VCU2_CAN1_toNidec] -> CSVCU2CAN1toNidec/1(CSVCU2CAN1toNidec)
  bus_selector20/1 -> FrIdcMaxtoNidec/1(FrIdcMaxtoNidec)  "<VOUTP_FrIdcMax_A>"
  [BOUTP_outputs] -> bus_selector20/1
  bus_selector21/1 -> FrIdcMintoNidec/1(FrIdcMintoNidec)  "<VOUTP_FrIdcMin_A>"
  [BOUTP_outputs] -> bus_selector21/1
  bus_selector22/1 -> FrTMTqReqtoNidec/1(FrTMTqReqtoNidec)  "<VOUTP_FrTMTqReq_Nm>"
  [BOUTP_outputs] -> bus_selector22/1
  Ground9/1 -> FrTorqMaxtoNidec/1(FrTorqMaxtoNidec)
  Ground10/1 -> FrTorqMintoNidec/1(FrTorqMintoNidec)
  bus_selector23/1 -> FrUdcMaxtoNidec/1(FrUdcMaxtoNidec)  "<VOUTP_FrUdcMax_V>"
  [BOUTP_outputs] -> bus_selector23/1
  bus_selector24/1 -> FrUdcMintoNidec/1(FrUdcMintoNidec)  "<VOUTP_FrUdcMin_V>"
  [BOUTP_outputs] -> bus_selector24/1
  RollingCounter_IfAction1/1 -> RCVCU2CAN1toNidec/1(RCVCU2CAN1toNidec)
  Constant4/1 -> RollingCounter_IfAction1/1
  bus_selector25/1 -> RrIdcMaxtoNidec/1(RrIdcMaxtoNidec)  "<VOUTP_RrIdcMax_A>"
  [BOUTP_outputs] -> bus_selector25/1
  bus_selector26/1 -> RrIdcMintoNidec/1(RrIdcMintoNidec)  "<VOUTP_RrIdcMin_A>"
  [BOUTP_outputs] -> bus_selector26/1
  bus_selector27/1 -> RrTMTqReqtoNidec/1(RrTMTqReqtoNidec)  "<VOUTP_RrTMTqReq_Nm>"
  [BOUTP_outputs] -> bus_selector27/1
  Ground11/1 -> RrTorqMaxtoNidec/1(RrTorqMaxtoNidec)
  Ground12/1 -> RrTorqMintoNidec/1(RrTorqMintoNidec)
  bus_selector28/1 -> RrUdcMaxtoNidec/1(RrUdcMaxtoNidec)  "<VOUTP_RrUdcMax_V>"
  [BOUTP_outputs] -> bus_selector28/1
  bus_selector29/1 -> RrUdcMintoNidec/1(RrUdcMintoNidec)  "<VOUTP_RrUdcMin_V>"
  [BOUTP_outputs] -> bus_selector29/1

== system halout/HAL_OUT/CAN3/FD3_VCU2_toNIDEC_Tx ==
  TxReq : Inport
  Chart : Stateflow chart  TreatAsAtomicUnit=on
  Constant : Constant  Value=C_TASK_5MS_S
  Constant3 : Constant  Value=CycleTime
  Data Type Conversion : DataTypeConversion  OutDataTypeStr=uint16
  Divide : Product  Inputs=*/
  Gain : Gain  Gain=0.001
  TxTrigger : Outport
  wires:
  Data Type Conversion/1 -> Chart/2(CycleCnt)
  Constant3/1 -> Gain/1
  Gain/1 -> Divide/1
  Chart/1(TxTrigger()) -> TxTrigger/1
  Divide/1 -> Data Type Conversion/1
  TxReq/1 -> Chart/1(TxReq)
  Constant/1 -> Divide/2

== system halout/HAL_OUT/CAN3/FD3_VCU5_0x155 ==
  BSCP_outputs : Inport  OutDataTypeStr=Bus: BSCP_outputs
  BOUTP_outputs : Inport  Port=2  OutDataTypeStr=Bus: BOUTP_outputs
  ActAPSPosn : Subsystem
  FrEDUSpd : Subsystem
  FrEDUSpdValid : Subsystem
  Ground{,1..3} (4 alike) : Ground
  RrEDUSpd : Subsystem
  RrEDUSpdValid : Subsystem
  bus_creator : BusCreator  Inputs=5  OutDataTypeStr=Bus: DT_CAN3_SG_FD3_VCU5  NonVirtualBus=on
  bus_selector : BusSelector  OutputSignals=VOUTP_ActAPSPosn_pct
  FD3_VCU5 : Outport
  wires:
  BSCP_outputs/1 -> [BSCP_outputs]
  BOUTP_outputs/1 -> [BOUTP_outputs]
  [CAN3_ActAPSPosn] -> bus_creator/1  "CAN3_ActAPSPosn"
  [CAN3_Fr_EDUSpd] -> bus_creator/2  "CAN3_Fr_EDUSpd"
  [CAN3_Fr_EDUSpdValid] -> bus_creator/3  "CAN3_Fr_EDUSpdValid"
  [CAN3_Rr_EDUSpd] -> bus_creator/4  "CAN3_Rr_EDUSpd"
  [CAN3_Rr_EDUSpdValid] -> bus_creator/5  "CAN3_Rr_EDUSpdValid"
  bus_creator/1 -> FD3_VCU5/1
  ActAPSPosn/1(CAN3_ActAPSPosn) -> [CAN3_ActAPSPosn]
  FrEDUSpd/1(CAN3_Fr_EDUSpd) -> [CAN3_Fr_EDUSpd]
  FrEDUSpdValid/1(CAN3_Fr_EDUSpdValid) -> [CAN3_Fr_EDUSpdValid]
  RrEDUSpd/1(CAN3_Rr_EDUSpd) -> [CAN3_Rr_EDUSpd]
  RrEDUSpdValid/1(CAN3_Rr_EDUSpdValid) -> [CAN3_Rr_EDUSpdValid]
  bus_selector/1 -> ActAPSPosn/1(ActAPSPosn)  "<VOUTP_ActAPSPosn_pct>"
  [BOUTP_outputs] -> bus_selector/1
  Ground/1 -> FrEDUSpd/1(FrEDUSpd)
  Ground1/1 -> FrEDUSpdValid/1(FrEDUSpdValid)
  Ground2/1 -> RrEDUSpd/1(RrEDUSpd)
  Ground3/1 -> RrEDUSpdValid/1(RrEDUSpdValid)

== system halout/HAL_OUT/CAN3/GW3_CE100_0_0x1C3 ==
  BSCP_outputs : Inport  OutDataTypeStr=Bus: BSCP_outputs
  BOUTP_outputs : Inport  Port=2  OutDataTypeStr=Bus: BOUTP_outputs
  CrashOutputSts : Subsystem
  DriverSeatBeltCmd : Subsystem
  Ground : Ground
  Ground1 : Ground
  VehSpeed : Subsystem
  bus_creator : BusCreator  Inputs=3  OutDataTypeStr=Bus: DT_CAN3_SG_GW3_CE100_0  NonVirtualBus=on
  bus_selector : BusSelector  OutputSignals=VOUTP_Vehspeed_kph
  GW3_CE100_0 : Outport
  wires:
  BSCP_outputs/1 -> [BSCP_outputs]
  BOUTP_outputs/1 -> [BOUTP_outputs]
  [CAN3_CrashOutputSts] -> bus_creator/1  "CAN3_CrashOutputSts"
  [CAN3_DriverSeatBeltCmd] -> bus_creator/2  "CAN3_DriverSeatBeltCmd"
  [CAN3_VehSpeed] -> bus_creator/3  "CAN3_VehSpeed"
  bus_creator/1 -> GW3_CE100_0/1
  CrashOutputSts/1(CAN3_CrashOutputSts) -> [CAN3_CrashOutputSts]
  DriverSeatBeltCmd/1(CAN3_DriverSeatBeltCmd) -> [CAN3_DriverSeatBeltCmd]
  VehSpeed/1(CAN3_VehSpeed) -> [CAN3_VehSpeed]
  Ground/1 -> CrashOutputSts/1(CrashOutputSts)
  Ground1/1 -> DriverSeatBeltCmd/1(DriverSeatBeltCmd)
  bus_selector/1 -> VehSpeed/1(VehSpeed)  "<VOUTP_Vehspeed_kph>"
  [BOUTP_outputs] -> bus_selector/1

== system halout/HAL_OUT/CAN4/FD4_C100_0_0x202 ==
  BSCP_outputs : Inport  OutDataTypeStr=Bus: BSCP_outputs
  BOUTP_outputs : Inport  Port=2  OutDataTypeStr=Bus: BOUTP_outputs
  FDCCHAEACEnDemandCmd : Subsystem
  bus_creator : BusCreator  Inputs=1  OutDataTypeStr=Bus: DT_CAN4_SG_FD4_C100_0  NonVirtualBus=on
  bus_selector : BusSelector  OutputSignals=VOUTP_EACEnDem_enum
  FD4_C100_0 : Outport
  wires:
  BSCP_outputs/1 -> [BSCP_outputs]
  BOUTP_outputs/1 -> [BOUTP_outputs]
  [CAN4_FDC_CHA_EACEnDemand_Cmd] -> bus_creator/1  "CAN4_FDC_CHA_EACEnDemand_Cmd"
  bus_creator/1 -> FD4_C100_0/1
  FDCCHAEACEnDemandCmd/1(CAN4_FDC_CHA_EACEnDemand_Cmd) -> [CAN4_FDC_CHA_EACEnDemand_Cmd]
  bus_selector/1 -> FDCCHAEACEnDemandCmd/1(FDCCHAEACEnDemandCmd)  "<VOUTP_EACEnDem_enum>"
  [BOUTP_outputs] -> bus_selector/1
